simulink model "custom_tank"  (R2024b)
settings: Solver=VariableStepAuto  StartTime=0.0  StopTime=1000  RelTol=1e-3
values from neighbouring files (symbols this model uses):
  A = 33    [Double_tank_parameters.m]    (also in Double_tank_parameters_non_disturbed.m)
  a = 0.16    [Double_tank_parameters.m]    (also in Double_tank_parameters_non_disturbed.m)
  Alin = [-alpha, 0; alpha, -alpha]    [Double_tank_parameters.m]    (also in Double_tank_parameters_non_disturbed.m)
  Blin = [beta; 0]    [Double_tank_parameters.m]    (also in Double_tank_parameters_non_disturbed.m)
  Clin = [0, 1]    [Double_tank_parameters.m]    (also in Double_tank_parameters_non_disturbed.m)
  Dlin = 0    [Double_tank_parameters.m]    (also in Double_tank_parameters_non_disturbed.m)
  fSamplingTime = 1/fSamplingFrequency    (= 0.0125)    [Double_tank_parameters.m]    (also in Double_tank_parameters_non_disturbed.m)
  g = 982    [Double_tank_parameters.m]    (also in Double_tank_parameters_non_disturbed.m)
  h = 15    [Double_tank_parameters.m]    (also in Double_tank_parameters_non_disturbed.m)
  h0 = 3.2    [Double_tank_parameters.m]    (also in Double_tank_parameters_non_disturbed.m)
  Kgain = Cd'*(Cd*P* Cd' + R2)    [Double_tank_parameters.m]    (also in Double_tank_parameters_non_disturbed.m)
  KgainC = Clin'*(Clin*PC*Clin' + R2)    [Double_tank_parameters_non_disturbed.m]
  N = Ed    [Double_tank_parameters.m]    (also in Double_tank_parameters_non_disturbed.m)
  p1 = polyfit(u0, fu0, 3)    [Double_tank_parameters.m]    (also in Double_tank_parameters_non_disturbed.m)
  Qd = R1    [Double_tank_parameters.m]    (also in Double_tank_parameters_non_disturbed.m)
  Rd = R2    (= 0.01)    [Double_tank_parameters.m]    (also in Double_tank_parameters_non_disturbed.m)
  u_h = r(n)    [Double_tank_parameters.m]    (also in Double_tank_parameters_non_disturbed.m)
undefined symbols (not defined in the file or in its folder): Ad, Bd, Cd, P
libraries: simulink x3
settings Model: Creator=beckl  LastModifiedBy=beckl

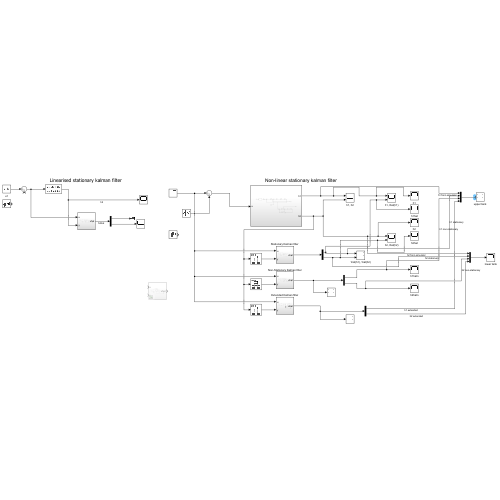
[thumbnail: Simulink's stored preview of the top-level diagram]
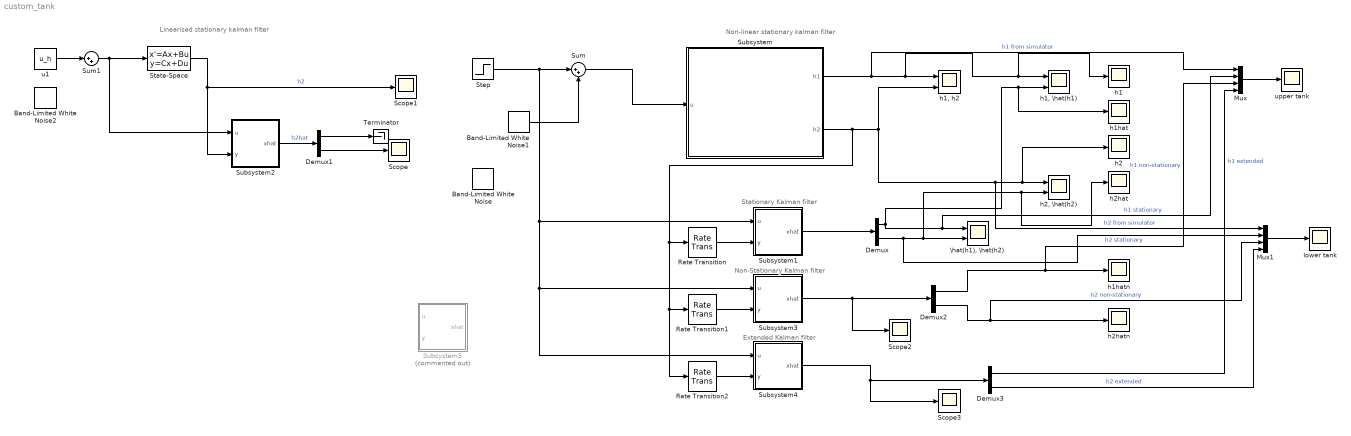
== system custom_tank ==
  note: Non-Stationary Kalman filter
  note: Extended Kalman filter
  note: Stationary Kalman filter
  note: Linearised stationary kalman filter
  note: Non-linear stationary kalman filter
  Band-Limited White Noise : simulink/Sources/Band-Limited White Noise  Cov=[0.1]  Ts=0.1  seed=[23341]
  Band-Limited White Noise1 : simulink/Sources/Band-Limited White Noise  Cov=[0.01]  Ts=fSamplingTime  seed=[23341]
  Band-Limited White Noise2 : simulink/Sources/Band-Limited White Noise  Cov=[0.1]  Ts=0.1  seed=[23341]
  Demux{,1..3} (4 alike) : Demux  Outputs=2
  Mux : Mux
  Mux1 : Mux
  Rate Transition : RateTransition  OutPortSampleTime=fSamplingTime
  Rate Transition1 : RateTransition  OutPortSampleTime=fSamplingTime
  Rate Transition2 : RateTransition  OutPortSampleTime=fSamplingTime
  Scope{,1..3} (4 alike) : Scope
  State-Space : StateSpace  A=Alin  B=Blin  C=Clin  D=Dlin  InitialCondition=0
  Step : Step  Time=100  After=u_h  SampleTime=0
  Subsystem : Subsystem
  Subsystem1 : Subsystem
  Subsystem2 : Subsystem
  Subsystem3 : Subsystem
  Subsystem4 : Subsystem
  Subsystem5 : Subsystem  Commented=on
  Sum : Sum  Inputs=|++
  Sum1 : Sum  Inputs=|++
  Terminator : Terminator
  "\\hat(h1), \\hat(h2)" : Scope  NumInputPorts=2
  h1 : Scope
  "h1, \\hat(h1)" : Scope  NumInputPorts=2
  "h1, h2" : Scope  NumInputPorts=2
  h1hat : Scope
  h1hatn : Scope
  h2 : Scope
  "h2, \\hat(h2)" : Scope  NumInputPorts=2
  h2hat : Scope
  h2hatn : Scope
  lower tank : Scope
  u1 : Constant  Value=u_h
  upper tank : Scope
  wires:
  Sum/1 -> Subsystem/1(u)
  Subsystem/1(h1) -> Mux/1, h1/1, "h1, \\hat(h1)"/1, "h1, h2"/1  "h1 from simulator"
  Subsystem/2(h2) -> Rate Transition2/1, Rate Transition1/1, Rate Transition/1, Mux1/1, h2/1, "h2, \\hat(h2)"/1, "h1, h2"/2  "h2 from simulator"
  Step/1 -> Subsystem4/1(u), Subsystem3/1(u), Subsystem1/1(u), Sum/1
  u1/1 -> Sum1/1
  Sum1/1 -> Subsystem2/1(u), State-Space/1
  Rate Transition/1 -> Subsystem1/2(y)
  Subsystem1/1(xhat) -> Demux/1
  Demux/1 -> Mux/2, "\\hat(h1), \\hat(h2)"/1, h1hat/1, "h1, \\hat(h1)"/2  "h1 stationary"
  Demux/2 -> Mux1/2, "\\hat(h1), \\hat(h2)"/2, h2hat/1, "h2, \\hat(h2)"/2  "h2 stationary"
  State-Space/1 -> Scope1/1, Subsystem2/2(y)  "h2"
  Subsystem2/1(xhat) -> Demux1/1  "h2hat"
  Demux1/1 -> Terminator/1
  Demux1/2 -> Scope/1
  Rate Transition1/1 -> Subsystem3/2(y)
  Subsystem3/1(xhat) -> Demux2/1, Scope2/1
  Demux2/2 -> Mux1/3, h2hatn/1  "h2 non-stationary"
  Demux2/1 -> Mux/3, h1hatn/1  "h1 non-stationary"
  Band-Limited White Noise1/1 -> Sum/2
  Rate Transition2/1 -> Subsystem4/2(y)
  Subsystem4/1(xhat) -> Demux3/1, Scope3/1
  Mux/1 -> upper tank/1
  Mux1/1 -> lower tank/1
  Demux3/1 -> Mux/4  "h1 extended"
  Demux3/2 -> Mux1/4  "h2 extended"

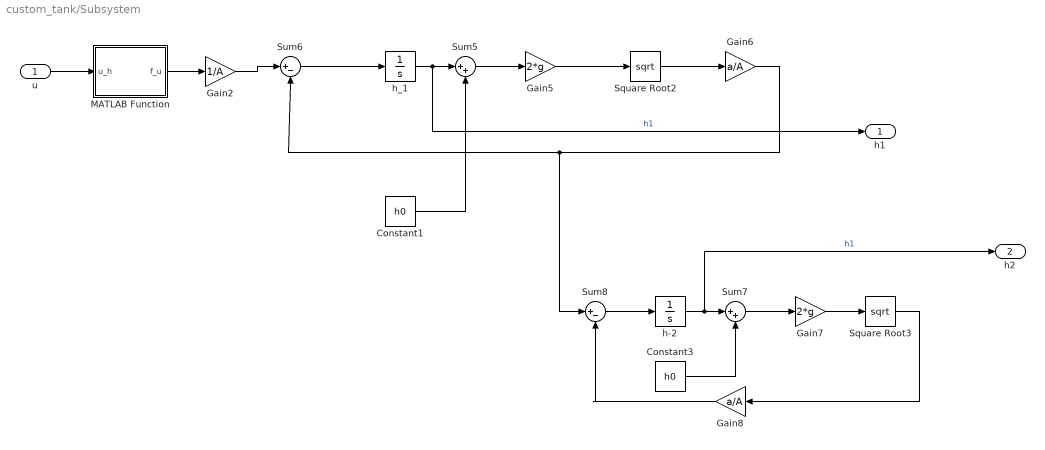
== system custom_tank/Subsystem ==
  u : Inport
  Constant1 : Constant  Value=h0
  Constant3 : Constant  Value=h0
  Gain2 : Gain  Gain=1/A
  Gain5 : Gain  Gain=2*g
  Gain6 : Gain  Gain=a/A
  Gain7 : Gain  Gain=2*g
  Gain8 : Gain  Gain=a/A
  MATLAB Function : MATLAB Function  TreatAsAtomicUnit=on
  Square Root2 : Sqrt
  Square Root3 : Sqrt
  Sum5 : Sum  Inputs=|++
  Sum6 : Sum  Inputs=|+-
  Sum7 : Sum  Inputs=|++
  Sum8 : Sum  Inputs=|+-
  h-2 : Integrator
  h_1 : Integrator
  h1 : Outport
  h2 : Outport  Port=2
  wires:
  Gain8/1 -> Sum8/2
  Sum6/1 -> h_1/1
  Gain7/1 -> Square Root3/1
  Sum8/1 -> h-2/1
  Gain6/1 -> Sum6/2, Sum8/1
  Constant3/1 -> Sum7/2
  h-2/1 -> h2/1, Sum7/1  "h1"
  Square Root3/1 -> Gain8/1
  MATLAB Function/1(f_u) -> Gain2/1
  Constant1/1 -> Sum5/2
  Sum7/1 -> Gain7/1
  Gain5/1 -> Square Root2/1
  Gain2/1 -> Sum6/1
  Sum5/1 -> Gain5/1
  h_1/1 -> h1/1, Sum5/1  "h1"
  Square Root2/1 -> Gain6/1
  u/1 -> MATLAB Function/1(u_h)

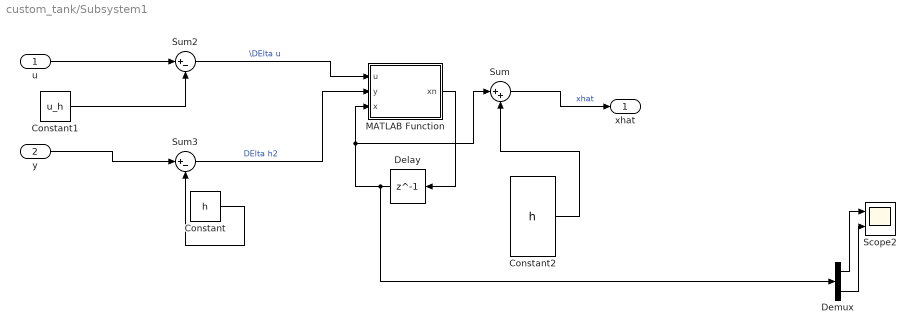
== system custom_tank/Subsystem1 ==
  u : Inport
  y : Inport  Port=2
  Constant : Constant  Value=h
  Constant1 : Constant  Value=u_h
  Constant2 : Constant  Value=h
  Delay : Delay  DelayLength=1  InitialCondition=[0;0]  SampleTime=fSamplingTime
  Demux : Demux  Outputs=2
  MATLAB Function : MATLAB Function  TreatAsAtomicUnit=on
  Scope2 : Scope  NumInputPorts=2
  Sum : Sum  Inputs=|++
  Sum2 : Sum  Inputs=|+-
  Sum3 : Sum  Inputs=|+-
  xhat : Outport
  wires:
  Constant/1 -> Sum3/2
  Constant1/1 -> Sum2/2
  u/1 -> Sum2/1
  y/1 -> Sum3/1
  Sum/1 -> xhat/1  "xhat"
  Sum3/1 -> MATLAB Function/2(y)  "DElta h2"
  Sum2/1 -> MATLAB Function/1(u)  "\\DElta u"
  Delay/1 -> Demux/1, Sum/1, MATLAB Function/3(x)
  Constant2/1 -> Sum/2
  MATLAB Function/1(xn) -> Delay/1
  Demux/2 -> Scope2/2
  Demux/1 -> Scope2/1

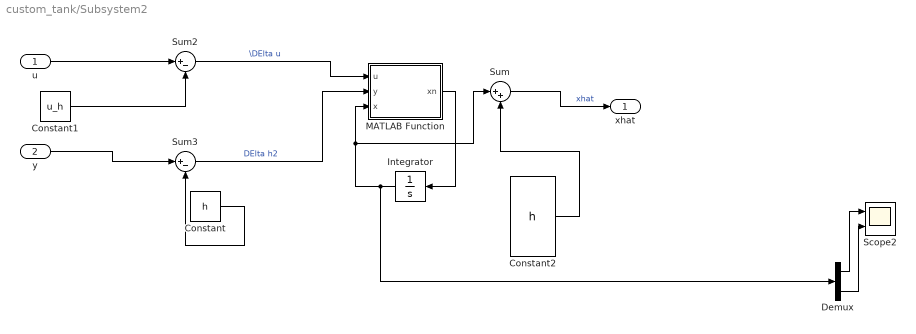
== system custom_tank/Subsystem2 ==
  u : Inport
  y : Inport  Port=2
  Constant : Constant  Value=h
  Constant1 : Constant  Value=u_h
  Constant2 : Constant  Value=h
  Demux : Demux  Outputs=2
  Integrator : Integrator
  MATLAB Function : MATLAB Function  TreatAsAtomicUnit=on
  Scope2 : Scope  NumInputPorts=2
  Sum : Sum  Inputs=|++
  Sum2 : Sum  Inputs=|+-
  Sum3 : Sum  Inputs=|+-
  xhat : Outport
  wires:
  Constant/1 -> Sum3/2
  u/1 -> Sum2/1
  y/1 -> Sum3/1
  Sum/1 -> xhat/1  "xhat"
  Sum3/1 -> MATLAB Function/2(y)  "DElta h2"
  Sum2/1 -> MATLAB Function/1(u)  "\\DElta u"
  Integrator/1 -> Demux/1, Sum/1, MATLAB Function/3(x)
  Constant2/1 -> Sum/2
  MATLAB Function/1(xn) -> Integrator/1
  Demux/2 -> Scope2/2
  Demux/1 -> Scope2/1
  Constant1/1 -> Sum2/2

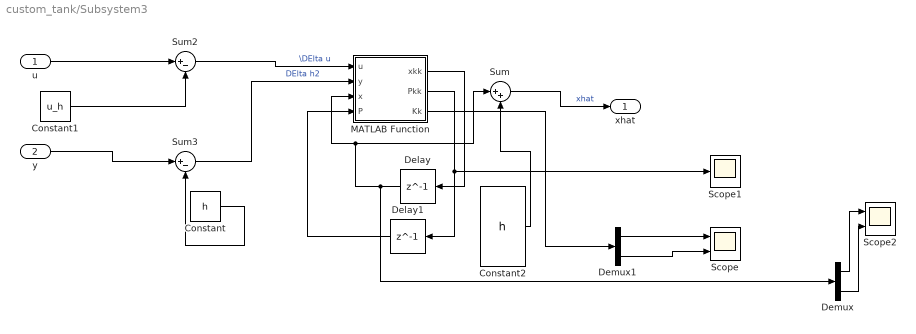
== system custom_tank/Subsystem3 ==
  u : Inport
  y : Inport  Port=2
  Constant : Constant  Value=h
  Constant1 : Constant  Value=u_h
  Constant2 : Constant  Value=h
  Delay : Delay  DelayLength=1  InitialCondition=[0;0]  SampleTime=fSamplingTime
  Delay1 : Delay  DelayLength=1  InitialCondition=P
  Demux : Demux  Outputs=2
  Demux1 : Demux  Outputs=2
  MATLAB Function : MATLAB Function  TreatAsAtomicUnit=on
  Scope : Scope  NumInputPorts=2
  Scope1 : Scope
  Scope2 : Scope  NumInputPorts=2
  Sum : Sum  Inputs=|++
  Sum2 : Sum  Inputs=|+-
  Sum3 : Sum  Inputs=|+-
  xhat : Outport
  wires:
  Constant/1 -> Sum3/2
  Constant1/1 -> Sum2/2
  u/1 -> Sum2/1
  y/1 -> Sum3/1
  Sum/1 -> xhat/1  "xhat"
  Sum3/1 -> MATLAB Function/2(y)  "DElta h2"
  Sum2/1 -> MATLAB Function/1(u)  "\\DElta u"
  Delay/1 -> Demux/1, Sum/1, MATLAB Function/3(x)
  Constant2/1 -> Sum/2
  MATLAB Function/1(xkk) -> Delay/1
  Demux/2 -> Scope2/2
  Demux/1 -> Scope2/1
  MATLAB Function/2(Pkk) -> Scope1/1, Delay1/1
  Delay1/1 -> MATLAB Function/4(P)
  MATLAB Function/3(Kk) -> Demux1/1
  Demux1/1 -> Scope/1
  Demux1/2 -> Scope/2

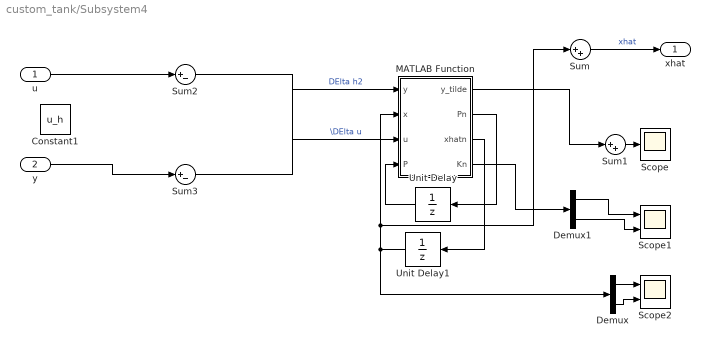
== system custom_tank/Subsystem4 ==
  u : Inport
  y : Inport  Port=2
  Constant1 : Constant  Value=u_h
  Demux : Demux  Outputs=2
  Demux1 : Demux  Outputs=2
  MATLAB Function : MATLAB Function  TreatAsAtomicUnit=on
  Scope : Scope
  Scope1 : Scope  NumInputPorts=2
  Scope2 : Scope  NumInputPorts=2
  Sum : Sum  Inputs=|++
  Sum1 : Sum  Inputs=|++
  Sum2 : Sum  Inputs=|+-
  Sum3 : Sum  Inputs=|+-
  Unit Delay : UnitDelay  InitialCondition=P  SampleTime=-1  HasFrameUpgradeWarning=on
  Unit Delay1 : UnitDelay  InitialCondition=[0;0]  SampleTime=-1  HasFrameUpgradeWarning=on
  xhat : Outport
  wires:
  u/1 -> Sum2/1
  y/1 -> Sum3/1
  Sum/1 -> xhat/1  "xhat"
  Sum3/1 -> MATLAB Function/1(y)  "DElta h2"
  Sum2/1 -> MATLAB Function/3(u)  "\\DElta u"
  Unit Delay1/1 -> MATLAB Function/2(x), Sum/1, Demux/1
  Demux/2 -> Scope2/2
  Demux/1 -> Scope2/1
  MATLAB Function/3(xhatn) -> Unit Delay1/1
  MATLAB Function/2(Pn) -> Unit Delay/1
  Unit Delay/1 -> MATLAB Function/4(P)
  Sum1/1 -> Scope/1
  MATLAB Function/1(y_tilde) -> Sum1/1
  Demux1/1 -> Scope1/1
  Demux1/2 -> Scope1/2
  MATLAB Function/4(Kn) -> Demux1/1

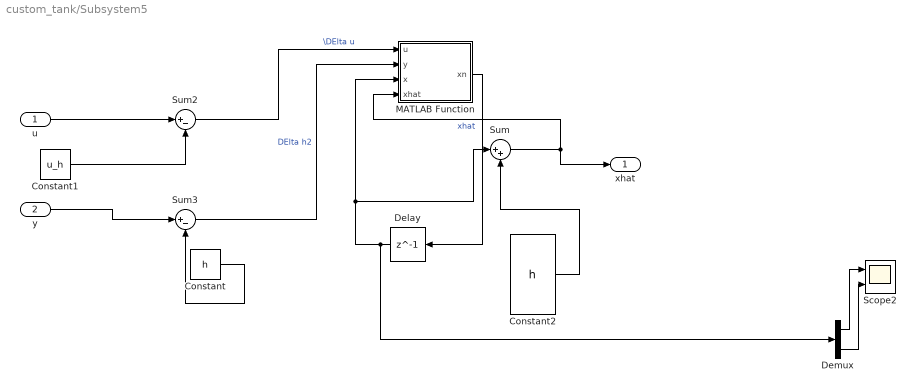
== system custom_tank/Subsystem5 ==
  u : Inport
  y : Inport  Port=2
  Constant : Constant  Value=h
  Constant1 : Constant  Value=u_h
  Constant2 : Constant  Value=h
  Delay : Delay  DelayLength=1  InitialCondition=[0;0]  SampleTime=fSamplingTime
  Demux : Demux  Outputs=2
  MATLAB Function : MATLAB Function  TreatAsAtomicUnit=on
  Scope2 : Scope  NumInputPorts=2
  Sum : Sum  Inputs=|++
  Sum2 : Sum  Inputs=|+-
  Sum3 : Sum  Inputs=|+-
  xhat : Outport
  wires:
  Constant/1 -> Sum3/2
  Constant1/1 -> Sum2/2
  u/1 -> Sum2/1
  y/1 -> Sum3/1
  Sum/1 -> MATLAB Function/4(xhat), xhat/1  "xhat"
  Sum3/1 -> MATLAB Function/2(y)  "DElta h2"
  Sum2/1 -> MATLAB Function/1(u)  "\\DElta u"
  Delay/1 -> Demux/1, Sum/1, MATLAB Function/3(x)
  Constant2/1 -> Sum/2
  MATLAB Function/1(xn) -> Delay/1
  Demux/2 -> Scope2/2
  Demux/1 -> Scope2/1

== matlab function custom_tank/Subsystem4/MATLAB Function ==
  data: y input; x input; y_tilde output; Pn output; u input; P input; p1 parameter; xhatn output; Qd parameter; Rd parameter; Kn output
function [y_tilde, Pn, xhatn, Kn] = fcn(y, x, u, P, p1, Qd, Rd)

fSamplingFrequency = 80;
fSamplingTime = 1/fSamplingFrequency;
A = 33; % 33 square centimetres
a = 0.16; % 0.16 square centimetres
T = 35; % 35 seconds time constant
K = 5; % metres per volt, motor gain
h = 12;
h0 = 3.2;
g = 982;


% Linearise around current point
alpha1 = g*a/(A*sqrt(2*g*(x(1)+h0)));
alpha2 = g*a/(A*sqrt(2*g*(x(2)+h0)));

A1 = [-alpha1, 0; alpha1, alpha2];
An = eye(size(A1)) + fSamplingTime*A1;
Cn = [0, 1];

% predict
q = p1(1)*u^3 + p1(2)*u^2 + p1(3)*u + p1(4);
xhatdot = [q/A - a/A*(sqrt(2*g*(x(1)+h0)));
    a/A * (sqrt(2*g*(x(1)+h0))) - a/A * (sqrt(2*g*(x(2)+h0)))];
xhatn = x + xhatdot.*fSamplingTime;
Pn = An * P * An' + Qd;

% update
y_tilde = y - Cn * xhatn;
S = Cn * Pn * Cn'+ Rd;
Kn = S\(Pn * Cn');
xhatn = xhatn + Kn*y_tilde;
Pn = (eye(size(An)) - Kn*Cn)*Pn;
y_tilde = y - Cn*xhatn;


% % ta in Y, Q, U, P,

% Från Joar och Ville
% function [xhatn, Pn] = fcn(u,y,xhat, Qd, Rd, N, Cd, u_h,Ad, h, fSamplingTime, fuprime, Bd, Kgain, P)
% % system constants
% A = 33; % 33 square centimetres
% a = 0.16; % 0.16 square centimetres
% h0 = 3.2;
% g = 982;
% 
 
% 
%     if u < 0.1 % when step input is given
%         %initialization
%         xhatn = [0;0];
%         yhat = 0;
%         Kn = Kgain;
%         Pn = P;
%         Adn = Ad;
%         Bdn = Bd;
% 
%     else
%         % firstly, convert absolute inputs/measurements to deviation
%         % variables
%         u_tilde = u-u_h;
%         y_tilde = y;
%         %update covariance matrix
%         Pn = Ad*P*Ad' + N*Qd*N';
% 
%         % update measurement
%         yhat = Cd*xhat;
%         residual = y_tilde - yhat;
% 
%         % update states
%         xhatn = Ad*xhat + Bd*u_tilde + Kgain*residual;
% 
%         % update kalman gain
%         Kn = (Cd*P*Cd' + Rd)\P*Cd';
% 
%         % make sure we have no complex numbers
%         h1_check = xhatn(1) + h;
%         h2_check = xhatn(2) + h;
%         if h1_check + h0 < 0.01; xhat(1) = 0.01 - h0 - h; end
%         if h2_check + h0 < 0.01; xhat(2) = 0.01 - h0 - h; end
% 
%         % recalculate alphas for A matrix
%         alpha1n = (a*g)/(A*sqrt(2*g*(xhat(1) + h0)));
%         alpha2n = (a*g)/(A*sqrt(2*g*(xhat(2) + h0)));
% 
%         % update discrete A matrix
%         Adn = [1 - fSamplingTime*alpha1n, 0; 
%             fSamplingTime*alpha1n, 1 - fSamplingTime*alpha2n];
% 
%         % update discrete B matrix using polyval
%         k_pump = polyval(fuprime, u_h);
%         Bdn = [fSamplingTime * (k_pump / A); 0];
% 
%         xhatn = Adn*xhatn + Bdn*u_h; 
% 
%     end
% end
% 
% % 
% % 
% % 
% % 
% % 
% % % Gamla grejer
% % % if x(1) < 0
% % %     x(1) = 0;
% % % end
% % % 
% % % if x(2) < 0
% % %     x(2) = 0;
% % % end
% % % 
% % % x1n = fu/A - a/A * sqrt(2*g*(x(1)+h0)); % for upper tank
% % % x2n = a/A * (sqrt(2*g*(x1n+h0)) - sqrt(2*g*(x(2)+h0))); % for lower tank
% % % 
% % % G = [x1n; x2n];
% % % y_tilde = y - G;
% % % 
% % % df1dx1 = -g*a/(A*sqrt(x(1)+h0));
% % % df1dx2 = 0;
% % % df2dx1 = g*a/(A*sqrt(x(1)+h0));
% % % df2dx2 = -g*a/(A*sqrt(x(2)+h0));
% % % c = g*a/(A*sqrt(x2n+h0));
% % % Ak = [df1dx1, df1dx2; df2dx1, df2dx2]+eye(2,2);
% % % Bk = [beta, 0]';
% % % Ck = [0, 1];
% % % Dk = 0;
% % % xk = [x1n; x2n];
% % % 
% % % Pk = Ak*P*Ak' + N*Qd*N';
% % % Kk = (Ck*Pk*Ck'+Rd)\(Pk*Ck');
% % % 
% % % xn = Ak*xk + Bk*u + Kk'*(y_tilde);

== matlab function custom_tank/Subsystem5/MATLAB Function ==
  data: u input; xn output; y input; x input; xhat input; p1 parameter
function xn = fcn(u,y,x,xhat,p1)
xn=[0;0];
u_h = u;
fSamplingFrequency = 50;
fSamplingTime = 1/fSamplingFrequency;
A = 33; % 33 square centimetres
a = 0.16; % 0.16 square centimetres
T = 35; % 35 seconds time constant
K = 5; % metres per volt, motor gain
h = 3;
h0 = 3.2;
g = 982;
alpha = g*a/(A*sqrt(2*g*(x(2)+h0)));
fuprime = p1(1)*3*u_h^2 + p1(2)*2*u_h + p1(3);
beta = fuprime/A;
Alin = [-alpha, 0; alpha, -alpha];
Blin = [beta; 0];
Clin = [0, 1];
Dlin = 0;

Ad = exp(Alin*fSamplingTime);
Bd = (exp(Alin*fSamplingTime))*fSamplingTime*Blin;
Cd = Clin;
Dd = Dlin;

R1 = eye(2)*0.01;
R2 = 0.01;
Qd = R1; % det var typ R1-matrisen i think
Rd = R2; % varians för noise

P = cov(x, xhat);
Kgain = Cd'*(Cd*P* Cd' + R2);


xn =Ad*x+Bd*u+Kgain*(y-Cd*x);

== matlab function custom_tank/Subsystem1/MATLAB Function ==
  data: u input; xn output; y input; x input; Ad parameter; Bd parameter; Cd parameter; Kgain parameter
function xn = fcn(u,y,x,Ad, Bd, Cd, Kgain)
xn=[0;0];
xn =Ad*x+Bd*u+Kgain*(y-Cd*x);

== matlab function custom_tank/Subsystem/MATLAB Function ==
  data: u_h input; f_u output; p1 parameter
function f_u = fcn(u_h,p1)
f_u  = polyval(p1, u_h);;

== matlab function custom_tank/Subsystem2/MATLAB Function ==
  data: u input; xn output; y input; x input; Alin parameter; Blin parameter; Clin parameter; KgainC parameter
function xn = fcn(u,y,x,Alin, Blin, Clin, KgainC)
xn=[0;0];
xn =Alin*x+Blin*u+KgainC*(y-Clin*x);

== matlab function custom_tank/Subsystem3/MATLAB Function ==
  data: u input; xkk output; y input; x input; Ad parameter; Bd parameter; Cd parameter; Qd parameter; Rd parameter; Pkk output; P input; Kk output; N parameter
function [xkk, Pkk, Kk] = fcn(u,y,x,Ad, Bd, Cd, Qd, Rd, P, N)
%xn =Ad*x+Bd*u+Kgain*(y-Cd*x); %stationary
%xn = Ad*x + Bd*u + N*v;
% Sk = 0
xk = Ad*x + Bd*u;
Pk = Ad*P*Ad' + N*Qd*N';
%Pk = cov(x, xk);

Kk = (Cd*Pk*Cd'+Rd)\(Pk*Cd');
y_tilde = y-Cd*xk;

xkk = xk + Kk*y_tilde;
Pkk = Pk - Kk*Cd*Pk;
